simulink model "power_motordrive_PMSM_FOC"  (R2021a)
settings: Solver=FixedStepDiscrete  StartTime=0.0  StopTime=0.8  RelTol=1e-3  EnableMultiTasking=on
PreLoadFcn:
  |  power_motordrive_PMSM_FOC_data
InitFcn:
  | power_motordrive_PMSM_FOC_data
values from neighbouring files (symbols this model uses):
  Rs = 0.02    [foc_model_Initialization.m]
undefined symbols (not defined in the file or in its folder): DiscIntNeverNeededParam, F, Fsw, gcbh, J, Ki_Ireg, Ki_wreg, Kp_Ireg, Kp_wreg, Limit_Ireg, Limit_wreg, p, sps_rtmsupport, Ts, Vdc_nom
libraries: simulink x6, spsStairGeneratorLib x2, spsSecondOrderFilterLib x2, spsPermanentMagnetSynchronousMachineLib x1, spsDCVoltageSourceLib x1, spsdq0toabcLib x1, spsabctodq0Lib x1, spsPowerdq0InstantaneousLib x1, spsThreePhaseVIMeasurementLib x1, spsTwoLevelConverterLib x1, spspowerguiLib x1
settings Model: SimulationMode=accelerator  Creator=The MathWorks, Inc.  LastModifiedBy=Hidayet
settings SolverCC: AlgebraicLoopSolver=TrustRegion
settings DataIOCC: SaveOutput=off  SignalLogging=off  DSMLogging=off  SaveTime=off  ReturnWorkspaceOutputs=off
settings DebuggingCC: SFMachineParentedDataDiag=warning

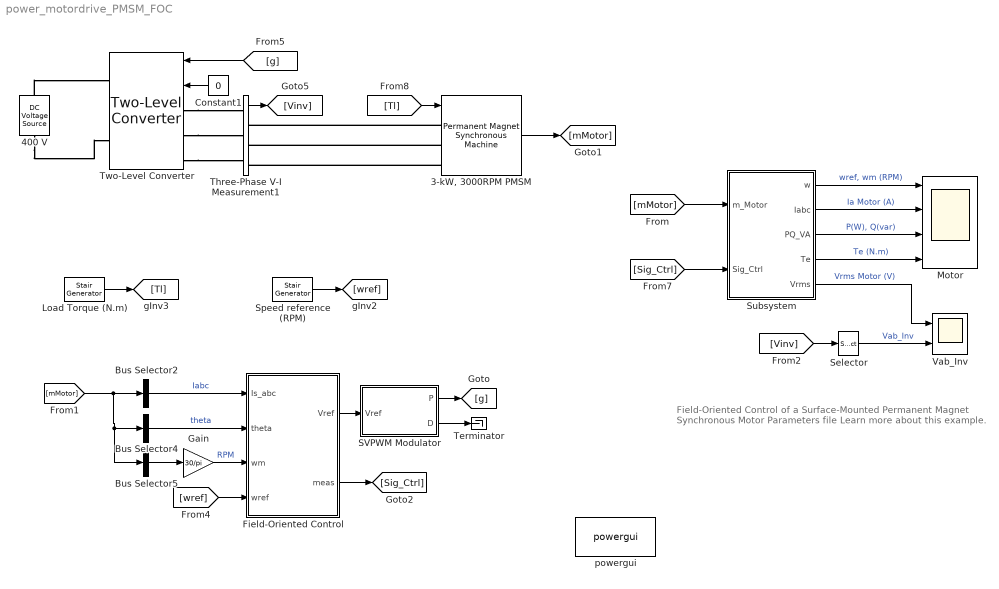
== system power_motordrive_PMSM_FOC ==
  note: Field-Oriented Control of a Surface-Mounted
      | Permanent Magnet Synchronous Motor
      | Parameters file
      |
      | Learn more about this example.
  "3-kW, 3000RPM PMSM" : spsPermanentMagnetSynchronousMachineLib/Permanent Magnet Synchronous Machine  NbPhases=3  FluxDistribution=Sinusoidal  RotorType=Round  MechanicalLoad=Torque Tm  PresetModel=No  ShowDetailedParameters=on  MeasurementBus=off  Resistance=Rs  Inductance=8.5e-3  dqInductances=[8.5e-3,8.5e-3]  La=La  MachineConstant=Flux linkage established by magnets (V.s)  Flux=lambda  VoltageCst=95.2245  TorqueCst=0.7875  Flat=120  Mechanical=[J F p 0]  PolePairs=4  InitialConditions=[0,0, 0,0]  InitialConditions5ph=[0 0 0 0 0 0]  RefAngle=90 degrees behind phase A axis (modified Park)  IterativeDiscreteModel=Trapezoidal robust  TsBlock=Ts  TsPowergui=0
  400 V : spsDCVoltageSourceLib/DC Voltage Source  Amplitude=Vdc_nom  Measurements=None
  Bus Selector2 : BusSelector  OutputSignals=Stator current is_a (A),Stator current is_b (A),Stator current is_c (A)  OutputAsBus=on
  Bus Selector4 : BusSelector  OutputSignals=Rotor angle thetam (rad)  OutputAsBus=on
  Bus Selector5 : BusSelector  OutputSignals=Rotor speed wm (rad/s)  OutputAsBus=on
  Constant1 : Constant  Value=0
  Field-Oriented Control : Subsystem  DialogController=POWERSYS.PowerSysDialog  LoadFcn=sps_rtmsupport('LoadFcn',gcbh);  StartFcn=sps_rtmsupport('StartFcn',gcbh);  StopFcn=sps_rtmsupport('StopFcn',gcbh);  mask(Field-Oriented Controller (FOC) of a PMSM drive){Kp_wreg=Kp_wreg, Ki_wreg=Ki_wreg, Limit_wreg=Limit_wreg, Kp_Ireg=Kp_Ireg, Ki_Ireg=Ki_Ireg, Limits_Ireg=Limit_Ireg, p=p, Ts=Ts}
      mask prompts: Kp_wreg "Proportional gain"; Ki_wreg "Integral gain"; Limit_wreg "Output (current) limit"; Kp_Ireg "Proportional gain"; Ki_Ireg "Integral gain"; Limits_Ireg "Output limit"; p "Number of pole pairs:"; Ts "Sample time (s)"
      settings: AttributesFormatString=\n  CopyFcn=sps_rtmsupport('CopyFcn',gcbh); powericon('psbloadfunction',gcbh,'gotofrom','UpdateGotoTag');  DeleteFcn=sps_rtmsupport('DeleteFcn',gcbh);  UndoDeleteFcn=sps_rtmsupport('UndoDeleteFcn',gcbh);  ModelCloseFcn=sps_rtmsupport('ModelCloseFcn',gcbh);  PreSaveFcn=sps_rtmsupport('PreSaveFcn',gcbh);  PostSaveFcn=sps_rtmsupport('PostSaveFcn',gcbh);  NameChangeFcn=sps_rtmsupport('NameChangeFcn',gcbh);  PreCopyFcn=sps_rtmsupport('PreCopyFcn',gcbh);  OpenFcn=sps_rtmsupport('OpenFcn',gcbh, [-1 2 -3 4 5 6 7 17 22 23]);  CloseFcn=sps_rtmsupport('CloseFcn',gcbh);  PreDeleteFcn=sps_rtmsupport('PreDeleteFcn',gcbh);
      mask Help: helpview(psbhelp);
      mask DialogControl Container11 Prompt: Control parameters
      mask DialogControl Container12 Prompt: Speed regulator
      mask DialogControl Container8 Prompt: Current regulators
  Gain : Gain  Gain=30/pi
  Load Torque (N.m) : spsStairGeneratorLib/Stair Generator  t=[0, 0.65]  e=[0,-8]  Ts=Ts
  Motor : Scope  NumInputPorts=4
  SVPWM Modulator : Subsystem  DialogController=POWERSYS.PowerSysDialog  LoadFcn=sps_rtmsupport('LoadFcn', gcbh);  StartFcn=sps_rtmsupport('StartFcn', gcbh);  StopFcn=sps_rtmsupport('StopFcn', gcbh);  mask(Unified PWM Modulator for a 2-level, 3-phase converter){PWMmethod=Space Vector PWM (SVPWM) with pulse averaging, Fsw=Fsw, Ts=Ts}
      mask prompts: PWMmethod "PWM method"; Fsw "Switching frequency (Hz):"; Ts "Sample time (s):"
      mask help:
      | Generate pulses for PWM-controlled two-level, three-phase power electronics converter with pulse averaging capability.
      |
      | The pulses generation can be perform using one of the following Pulse-Width Modulation (PWM) methods:
      | 1. Sinusoidal PWM (SPWM)
      | 2. Sinusoidal PWM (SPWM) with pulse averaging
      | 3. Space Vector PWM (SVPWM)
      | 4. Space Vector PWM (SVPWM) with pulse averaging
      | 5. 30 degrees discontinuous PWM
      |
      | When a PWM method with pulse averaging is selected, the output pulses are averaged over one sample time. (Pulses value will range from 0 to 1)
      mask init:
      | switch PWMmethod
      |     case 1 % SPWM
      |         ZeroOrderHold_Ts=-1;
      |         Pavg=0;
      |     case 2 % SPWM with pulse averaging
      |         ZeroOrderHold_Ts=-1;
      |         Pavg=1;
      |     case 3  % SVPWM
      |         ZeroOrderHold_Ts=-1;
      |         Pavg=0;
      |     case 4  % SVPWM with pulse averaging
      |         ZeroOrderHold_Ts=-1;
      |         Pavg=1;
      |     case 5  % 30 degrees discontinuous PWM
      |         ZeroOrderHold_Ts=1/Fsw/2;
      |         Pavg=0;
      | end
      settings: CopyFcn=sps_rtmsupport('CopyFcn', gcbh);  DeleteFcn=sps_rtmsupport('DeleteFcn', gcbh);  UndoDeleteFcn=sps_rtmsupport('UndoDeleteFcn', gcbh);  ModelCloseFcn=sps_rtmsupport('ModelCloseFcn', gcbh);  PreSaveFcn=sps_rtmsupport('PreSaveFcn', gcbh);  PostSaveFcn=sps_rtmsupport('PostSaveFcn', gcbh);  NameChangeFcn=sps_rtmsupport('NameChangeFcn', gcbh);  PreCopyFcn=sps_rtmsupport('PreCopyFcn', gcbh);  OpenFcn=sps_rtmsupport('OpenFcn', gcbh, [1]);  CloseFcn=sps_rtmsupport('CloseFcn', gcbh);  PreDeleteFcn=sps_rtmsupport('PreDeleteFcn', gcbh);
      mask TypeOptions PWMmethod: Sinusoidal PWM (SPWM) | Sinusoidal PWM (SPWM) wirh pulse averaging | Space Vector PWM (SVPWM) | Space Vector PWM (SVPWM) with pulse averaging | 30 degrees discontinuous PWM
  Selector : Selector  InputPortWidth=3  IndexOptions=Index vector (dialog)  Indices=1  OutputSizes=1
  Speed reference (RPM) : spsStairGeneratorLib/Stair Generator  t=[0, 0.25]  e=[2000, -2800]  Ts=Ts
  Subsystem : Subsystem
  Terminator : Terminator
  Three-Phase V-I Measurement1 : spsThreePhaseVIMeasurementLib/Three-Phase V-I Measurement  VoltageMeasurement=phase-to-phase  SetLabelV=off  LabelV=Vabc  Vpu=off  VpuLL=off  CurrentMeasurement=no  SetLabelI=off  LabelI=Iabc  Ipu=off  Pbase=100e6  Vbase=500e3  OutputType=Complex  PhasorSimulation=off  PSBequivalent=0
  Two-Level Converter : spsTwoLevelConverterLib/Two-Level Converter  ModelType=Switching function  Ron=1e-3  Rs=1e6  Cs=inf  Vforward=[0,0]  Ron_Diode=1e-3  Rs_Diode=1e6  Cs_Diode=inf  Vf_Diode=0  Rs_CurrentSource=inf
      settings: SourceProductBaseCode=PS
  Vab_Inv : Scope  NumInputPorts=2
  powergui : spspowerguiLib/powergui  Priority=1  SimulationMode=Discrete  SampleTime=Ts  frequency=60  Iterations=50  frequencyindice=0  Pbase=100e6  ErrMax=1e-4  UnitsV=kV  UnitsW=MW  buscounter=0  FunctionMessages=off  echomessages=off  EnableUseOfTLC=off  CurrentSourceSwitches=off  DisableSnubberDevices=off  DisableRonSwitches=off  DisableVfSwitches=off  DisplayEquations=off  AutomaticDiscreteSolvers=off  SolverType=Tustin/Backward Euler (TBE)  Interpol=off  ExternalGateDelay=off  methode=off  Ts=100  x0status=blocks  SPID=on  SwTol=0  HookPort=off  NonlinearTolerance=1e-4  nMaxIteration=100  ContinueOnMaxIteration=off  RestoreLinks=warning  ResistiveCurrentMeasurement=off  Frange=[0:2:500]  Ylog=off  Xlog=on  ShowGrid=off  save=off  variable=ZData  structure=Scope_Compare  ZoomFFT=off  StartTime=0.75  cycles=1  DisplayStyle=1  fundamental=100  FreqAxis=off  MaxFrequency=25000  frequencyindicesteady=1  RmsSteady=1  display=off
  wires:
  Subsystem/5(Vrms) -> Vab_Inv/1  "Vrms Motor (V)"
  Selector/1 -> Vab_Inv/2  "Vab_Inv"
  Subsystem/4(Te) -> Motor/4  "Te (N.m)"
  Field-Oriented Control/1(Vref) -> SVPWM Modulator/1(Vref)
  Field-Oriented Control/2(meas) -> [Sig_Ctrl]
  [Vinv] -> Selector/1
  Subsystem/1(w) -> Motor/1  "wref, wm (RPM)"
  Subsystem/2(Iabc) -> Motor/2  "Ia Motor (A)"
  Subsystem/3(PQ_VA) -> Motor/3  "P(W), Q(var)"
  [mMotor] -> Subsystem/1(m_Motor)
  [Sig_Ctrl] -> Subsystem/2(Sig_Ctrl)
  [wref] -> Field-Oriented Control/4(wref)
  [mMotor] -> Bus Selector2/1, Bus Selector4/1, Bus Selector5/1
  Bus Selector2/1 -> Field-Oriented Control/1(Is_abc)  "Iabc"
  "3-kW, 3000RPM PMSM"/1 -> [mMotor]
  Constant1/1 -> Two-Level Converter/2
  Three-Phase V-I Measurement1/1 -> [Vinv]
  [Tl] -> "3-kW, 3000RPM PMSM"/1
  [g] -> Two-Level Converter/1
  Speed reference (RPM)/1 -> [wref]
  Load Torque (N.m)/1 -> [Tl]
  Bus Selector5/1 -> Gain/1
  Gain/1 -> Field-Oriented Control/3(wm)  "RPM"
  Bus Selector4/1 -> Field-Oriented Control/2(theta)  "theta"
  SVPWM Modulator/1(P) -> [g]
  SVPWM Modulator/2(D) -> Terminator/1
  connections:
  400 V/RConn1 -- Two-Level Converter/RConn1
  "3-kW, 3000RPM PMSM"/LConn1 -- Three-Phase V-I Measurement1/RConn1
  Two-Level Converter/LConn3 -- Three-Phase V-I Measurement1/LConn3
  "3-kW, 3000RPM PMSM"/LConn2 -- Three-Phase V-I Measurement1/RConn2
  Two-Level Converter/LConn1 -- Three-Phase V-I Measurement1/LConn1
  Two-Level Converter/LConn2 -- Three-Phase V-I Measurement1/LConn2
  400 V/LConn1 -- Two-Level Converter/RConn2
  "3-kW, 3000RPM PMSM"/LConn3 -- Three-Phase V-I Measurement1/RConn3

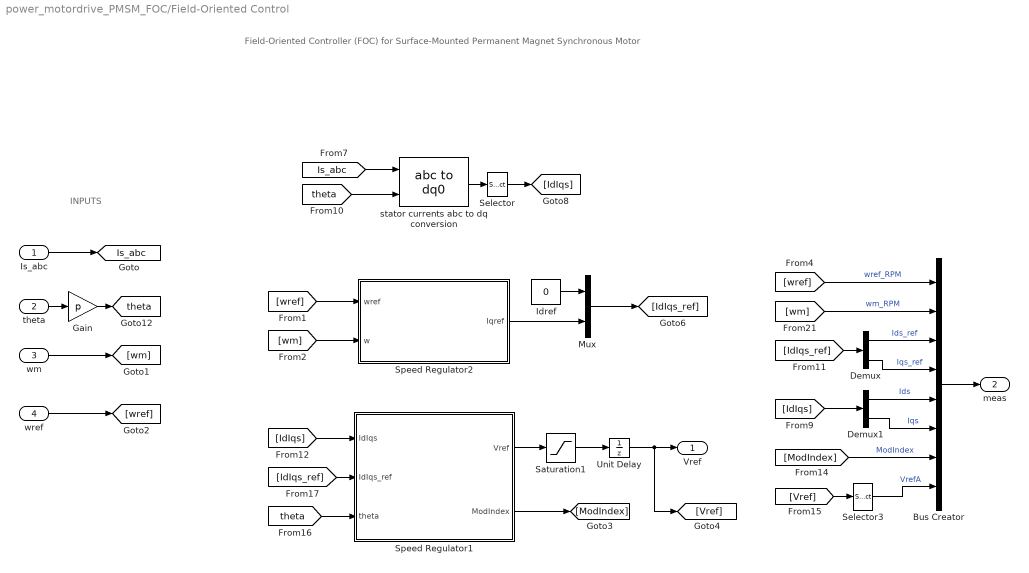
== system power_motordrive_PMSM_FOC/Field-Oriented Control ==
  note: INPUTS
  note: Field-Oriented Controller (FOC)
      | for
      | Surface-Mounted Permanent Magnet Synchronous Motor
  Is_abc : Inport  PortDimensions=3
  theta : Inport  Port=2  PortDimensions=1
  wm : Inport  Port=3  PortDimensions=1
  wref : Inport  Port=4  PortDimensions=1
  Bus Creator : BusCreator  Inputs=8
  Demux : Demux  Outputs=2
  Demux1 : Demux  Outputs=2
  Gain : Gain  Gain=p
  Idref : Constant  Value=0  SampleTime=Ts
  Mux : Mux  Inputs=2
  Saturation1 : Saturate  UpperLimit=2/sqrt(3)  LowerLimit=-2/sqrt(3)
  Selector : Selector  InputPortWidth=3  IndexOptions=Index vector (dialog)  Indices=[1 2]  OutputSizes=1
  Selector3 : Selector  InputPortWidth=3  IndexOptions=Index vector (dialog)  Indices=1  OutputSizes=1
  Speed Regulator1 : Subsystem  DialogController=POWERSYS.PowerSysDialog  mask(Current Regulators){Kp=Kp_Ireg, Ki=Ki_Ireg, Limits=Limits_Ireg, Init=0, Ts=Ts}
      mask prompts: Kp "Proportional gain (Kp):"; Ki "Integral gain (Ki):"; Limits "Output limits"; Init "Output initial value:"; Ts "Sample time:"
      mask help: This block implements two current regulators (Id & Iq) using anti-windup PI controllers.
      mask Display: disp('Current\nRegulators');
  Speed Regulator2 : Subsystem  DialogController=POWERSYS.PowerSysDialog  mask(Speed Regulator){Kp=Kp_wreg, Ki=Ki_wreg, Limit_wreg=Limit_wreg, Init=0, Ts=Ts}
      mask prompts: Kp "Proportional gain (Kp):"; Ki "Integral gain (Ki):"; Limit_wreg "Output limits"; Init "Output initial value:"; Ts "Sample time:"
      mask help: This block implements a speed regulator using an ant-windup PI controller.
      mask Display: disp('Speed\nRegulator');
  Unit Delay : UnitDelay  SampleTime=-1  HasFrameUpgradeWarning=on
  stator currents abc to dq conversion : spsabctodq0Lib/abc to dq0  Alignment=90 degrees behind phase A axis
  Vref : Outport  PortDimensions=3
  meas : Outport  Port=2
  tag scope: Is_abc=global, theta=global
  wires:
  Gain/1 -> [theta]
  Selector3/1 -> Bus Creator/8  "VrefA"
  [ModIndex] -> Bus Creator/7  "ModIndex"
  Mux/1 -> [IdIqs_ref]
  [IdIqs_ref] -> Speed Regulator1/2(IdIqs_ref)
  Idref/1 -> Mux/1
  Speed Regulator2/1(Iqref) -> Mux/2
  wref/1 -> [wref]
  theta/1 -> Gain/1
  Saturation1/1 -> Unit Delay/1
  [Vref] -> Selector3/1
  Speed Regulator1/2(ModIndex) -> [ModIndex]
  [IdIqs] -> Demux1/1
  Demux1/2 -> Bus Creator/6  "Iqs"
  Demux1/1 -> Bus Creator/5  "Ids"
  [IdIqs_ref] -> Demux/1
  Demux/2 -> Bus Creator/4  "Iqs_ref"
  Demux/1 -> Bus Creator/3  "Ids_ref"
  [wm] -> Bus Creator/2  "wm_RPM"
  [wref] -> Bus Creator/1  "wref_RPM"
  [IdIqs] -> Speed Regulator1/1(IdIqs)
  [theta] -> Speed Regulator1/3(theta)
  Is_abc/1 -> [Is_abc]
  Speed Regulator1/1(Vref) -> Saturation1/1
  stator currents abc to dq conversion/1 -> Selector/1
  [theta] -> stator currents abc to dq conversion/2
  [wm] -> Speed Regulator2/2(w)
  [wref] -> Speed Regulator2/1(wref)
  [Is_abc] -> stator currents abc to dq conversion/1
  Selector/1 -> [IdIqs]
  Unit Delay/1 -> [Vref], Vref/1
  Bus Creator/1 -> meas/1
  wm/1 -> [wm]

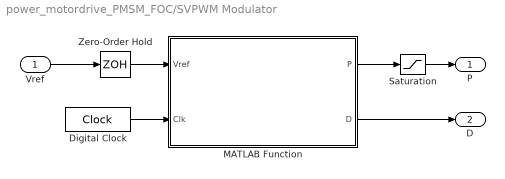
== system power_motordrive_PMSM_FOC/SVPWM Modulator ==
  Vref : Inport  PortDimensions=3  SampleTime=Ts
  Digital Clock : DigitalClock  SampleTime=Ts
  MATLAB Function : MATLAB Function  TreatAsAtomicUnit=on
  Saturation : Saturate  UpperLimit=1  LowerLimit=0
  Zero-Order Hold : ZeroOrderHold  SampleTime=ZeroOrderHold_Ts
  P : Outport  PortDimensions=6  SampleTime=Ts  VectorParamsAs1DForOutWhenUnconnected=off
  D : Outport  Port=2  PortDimensions=3  SampleTime=Ts  VectorParamsAs1DForOutWhenUnconnected=off
  wires:
  MATLAB Function/2(D) -> D/1
  MATLAB Function/1(P) -> Saturation/1
  Vref/1 -> Zero-Order Hold/1
  Saturation/1 -> P/1
  Digital Clock/1 -> MATLAB Function/2(Clk)
  Zero-Order Hold/1 -> MATLAB Function/1(Vref)

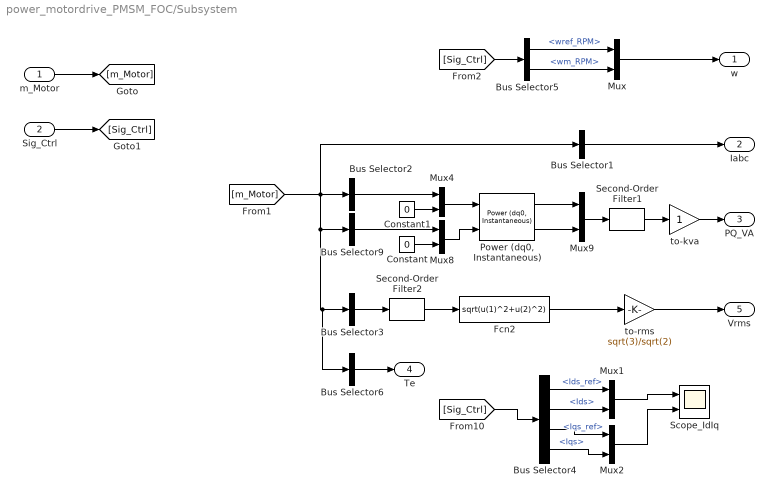
== system power_motordrive_PMSM_FOC/Subsystem ==
  m_Motor : Inport
  Sig_Ctrl : Inport  Port=2
  Bus Selector1 : BusSelector  OutputSignals=Stator current is_a (A),Stator current is_b (A),Stator current is_c (A)  OutputAsBus=on
  Bus Selector2 : BusSelector  OutputSignals=Stator voltage Vs_d (V),Stator voltage Vs_q (V)  OutputAsBus=on
  Bus Selector3 : BusSelector  OutputSignals=Stator voltage Vs_d (V),Stator voltage Vs_q (V)  OutputAsBus=on
  Bus Selector4 : BusSelector  OutputSignals=Ids_ref,Ids,Iqs_ref,Iqs
  Bus Selector5 : BusSelector  OutputSignals=wref_RPM,wm_RPM
  Bus Selector6 : BusSelector  OutputSignals=Electromagnetic torque Te (N*m)  OutputAsBus=on
  Bus Selector9 : BusSelector  OutputSignals=Stator current is_d (A),Stator current is_q (A)  OutputAsBus=on
  Constant : Constant  Value=0
  Constant1 : Constant  Value=0
  Fcn2 : Fcn  Expr=sqrt(u(1)^2+u(2)^2)
  Mux{,1..2,9} (4 alike) : Mux  Inputs=2
  Mux4 : Mux  Inputs=[2, 1]
  Mux8 : Mux  Inputs=[2, 1]
  "Power (dq0, Instantaneous)" : spsPowerdq0InstantaneousLib/Power (dq0, Instantaneous)
      settings: SourceProductBaseCode=PS
  Scope_IdIq : Scope  NumInputPorts=2
  Second-Order Filter1 : spsSecondOrderFilterLib/Second-Order Filter  FilterType=Lowpass  Fo=80  Zeta=1  Ts=Ts  Initialize=off  Vac_Init="[0,  0,  60]"  Vdc_Init=0  PlotResponse=off  FreqRange=[0, 500, 1]
      settings: SourceProductBaseCode=PS
  Second-Order Filter2 : spsSecondOrderFilterLib/Second-Order Filter  FilterType=Lowpass  Fo=120  Zeta=1  Ts=Ts  Initialize=off  Vac_Init="[0,  0,  60]"  Vdc_Init=0  PlotResponse=off  FreqRange=[0, 500, 1]
      settings: SourceProductBaseCode=PS
  to-kva : Gain
  to-rms : Gain  Gain=sqrt(3)/sqrt(2)
  w : Outport
  Iabc : Outport  Port=2
  PQ_VA : Outport  Port=3
  Te : Outport  Port=4
  Vrms : Outport  Port=5
  wires:
  Bus Selector6/1 -> Te/1
  Mux2/1 -> Scope_IdIq/2
  Mux1/1 -> Scope_IdIq/1
  Bus Selector4/4 -> Mux2/2  "<Iqs>"
  Bus Selector4/3 -> Mux2/1  "<Iqs_ref>"
  Bus Selector4/2 -> Mux1/2  "<Ids>"
  Bus Selector4/1 -> Mux1/1  "<Ids_ref>"
  Bus Selector1/1 -> Iabc/1
  Bus Selector5/2 -> Mux/2  "<wm_RPM>"
  Bus Selector5/1 -> Mux/1  "<wref_RPM>"
  [Sig_Ctrl] -> Bus Selector5/1
  [Sig_Ctrl] -> Bus Selector4/1
  Mux/1 -> w/1
  Mux8/1 -> "Power (dq0, Instantaneous)"/2
  Second-Order Filter2/1 -> Fcn2/1
  Fcn2/1 -> to-rms/1
  to-kva/1 -> PQ_VA/1
  to-rms/1 -> Vrms/1
  Second-Order Filter1/1 -> to-kva/1
  Mux9/1 -> Second-Order Filter1/1
  "Power (dq0, Instantaneous)"/1 -> Mux9/1
  Bus Selector2/1 -> Mux4/1
  "Power (dq0, Instantaneous)"/2 -> Mux9/2
  Constant/1 -> Mux8/2
  Bus Selector9/1 -> Mux8/1
  Constant1/1 -> Mux4/2
  Bus Selector3/1 -> Second-Order Filter2/1
  Mux4/1 -> "Power (dq0, Instantaneous)"/1
  [m_Motor] -> Bus Selector3/1, Bus Selector6/1, Bus Selector9/1, Bus Selector1/1, Bus Selector2/1
  m_Motor/1 -> [m_Motor]
  Sig_Ctrl/1 -> [Sig_Ctrl]

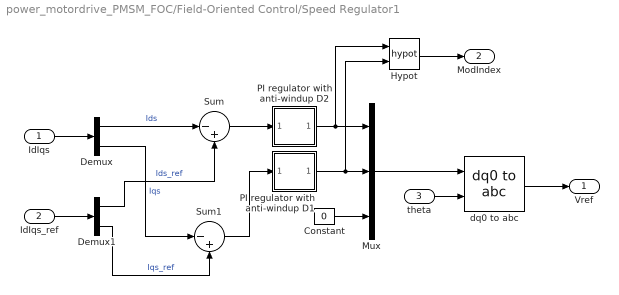
== system power_motordrive_PMSM_FOC/Field-Oriented Control/Speed Regulator1 ==
  IdIqs : Inport  PortDimensions=2
  IdIqs_ref : Inport  Port=2  PortDimensions=2
  theta : Inport  Port=3  PortDimensions=1
  Constant : Constant  Value=0
  Demux : Demux  Outputs=2
  Demux1 : Demux  Outputs=2
  Hypot : Math  Operator=hypot  SaturateOnIntegerOverflow=on
  Mux : Mux  Inputs=3
  PI regulator with anti-windup D1 : Subsystem  DialogController=POWERSYS.PowerSysDialog  mask(Discrete PI Controller){Kp=Kp, Ki=Ki, Par_Limits=[Limits -Limits], Init=0, Ts=Ts}
      mask prompts: Kp "Proportional gain (Kp):"; Ki "Integral gain (Ki):"; Par_Limits "Output limits: [ Upper   Lower ]"; Init "Output initial value:"; Ts "Sample time:"
      mask help: This block implements a discrete PI controller.
      mask init:
      | UpperLimit=Par_Limits(1);
      | LowerLimit=Par_Limits(2);
      | power_initmask();
      mask Help: This block is part of a subset of blocks in the Extras library that does not have documentation associated with it, other than the block mask description.
      mask Display: disp('PI');
  PI regulator with anti-windup D2 : Subsystem  DialogController=POWERSYS.PowerSysDialog  mask(Discrete PI Controller){Kp=Kp, Ki=Ki, Par_Limits=[Limits -Limits], Init=0, Ts=Ts}
      mask prompts: Kp "Proportional gain (Kp):"; Ki "Integral gain (Ki):"; Par_Limits "Output limits: [ Upper   Lower ]"; Init "Output initial value:"; Ts "Sample time:"
      mask help: This block implements a discrete PI controller.
      mask init:
      | UpperLimit=Par_Limits(1);
      | LowerLimit=Par_Limits(2);
      | power_initmask();
      mask Help: This block is part of a subset of blocks in the Extras library that does not have documentation associated with it, other than the block mask description.
      mask Display: disp('PI');
  Sum : Sum  Inputs=|-+
  Sum1 : Sum  Inputs=|-+
  dq0 to abc : spsdq0toabcLib/dq0 to abc  Alignment=90 degrees behind phase A axis
  Vref : Outport
  ModIndex : Outport  Port=2
  wires:
  Hypot/1 -> ModIndex/1
  dq0 to abc/1 -> Vref/1
  Demux1/1 -> Sum/2  "Ids_ref"
  Demux/1 -> Sum/1  "Ids"
  Demux1/2 -> Sum1/2  "Iqs_ref"
  IdIqs_ref/1 -> Demux1/1
  IdIqs/1 -> Demux/1
  PI regulator with anti-windup D2/1(Out) -> Mux/1, Hypot/1
  Sum/1 -> PI regulator with anti-windup D2/1(Error)
  PI regulator with anti-windup D1/1(Out) -> Mux/2, Hypot/2
  Constant/1 -> Mux/3
  Sum1/1 -> PI regulator with anti-windup D1/1(Error)
  Mux/1 -> dq0 to abc/1
  theta/1 -> dq0 to abc/2
  Demux/2 -> Sum1/1  "Iqs"

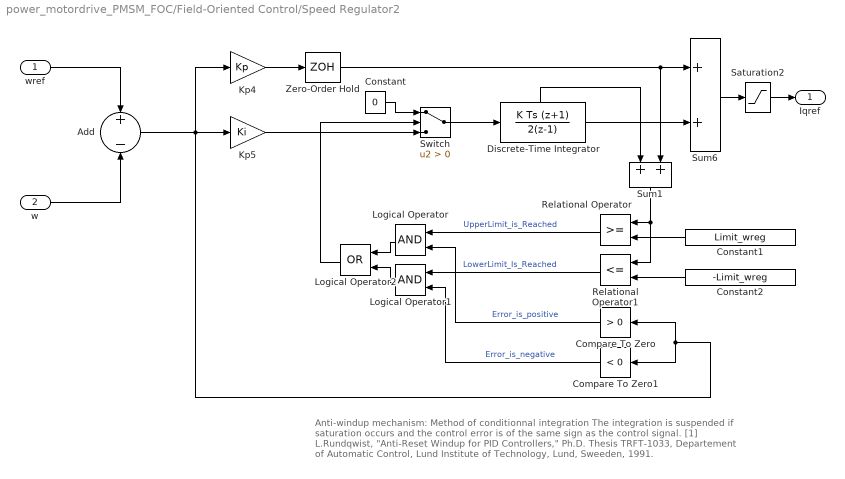
== system power_motordrive_PMSM_FOC/Field-Oriented Control/Speed Regulator2 ==
  note: Anti-windup mechanism: Method of conditionnal integration
      |
      | The integration is suspended if saturation occurs and the
      | control error is of the same sign as the control signal.
      |
      | [1] L.Rundqwist, "Anti-Reset Windup for PID Controllers," Ph.D. Thesis TRFT-1033,
      | Departement of Automatic Control, Lund Institute of Technology, Lund, Sweeden, 1991.
  wref : Inport  PortDimensions=1
  w : Inport  Port=2  PortDimensions=1
  Add : Sum  Inputs=+|-
  Compare To Zero : simulink/Logic and Bit Operations/Compare To Zero  relop=>  OutDataTypeStr=uint8  ZeroCross=off
  Compare To Zero1 : simulink/Logic and Bit Operations/Compare To Zero  relop=<  OutDataTypeStr=uint8  ZeroCross=off
  Constant : Constant  Value=0
  Constant1 : Constant  Value=Limit_wreg
  Constant2 : Constant  Value=-Limit_wreg
  Discrete-Time Integrator : DiscreteIntegrator  IntegratorMethod=Integration: Trapezoidal  InitialCondition=Init  SampleTime=Ts  LimitOutput=on  UpperSaturationLimit=Limit_wreg  LowerSaturationLimit=-Limit_wreg  ShowStatePort=on  ICPrevOutput=DiscIntNeverNeededParam  ICPrevScaledInput=DiscIntNeverNeededParam
  Kp4 : Gain  Gain=Kp  SaturateOnIntegerOverflow=on  SampleTime=Ts  OutDataTypeStr=Inherit: Same as input  ParamDataTypeStr=Inherit: Same as input
  Kp5 : Gain  Gain=Ki  SaturateOnIntegerOverflow=on  SampleTime=Ts  OutDataTypeStr=Inherit: Same as input  ParamDataTypeStr=Inherit: Same as input
  Logical Operator : Logic  AllPortsSameDT=off  OutDataTypeStr=boolean
  Logical Operator1 : Logic  AllPortsSameDT=off  OutDataTypeStr=boolean
  Logical Operator2 : Logic  Operator=OR  AllPortsSameDT=off  OutDataTypeStr=boolean
  Relational Operator : RelationalOperator  OutDataTypeStr=boolean  RndMeth=Nearest
  Relational Operator1 : RelationalOperator  Operator=<=  OutDataTypeStr=boolean  RndMeth=Nearest
  Saturation2 : Saturate  UpperLimit=Limit_wreg  LowerLimit=-Limit_wreg  SampleTime=Ts
  Sum1 : Sum  InputSameDT=on  SaturateOnIntegerOverflow=on  SampleTime=Ts  OutDataTypeStr=Inherit: Same as first input
  Sum6 : Sum  InputSameDT=on  SaturateOnIntegerOverflow=on  SampleTime=Ts  OutDataTypeStr=Inherit: Same as first input
  Switch : Switch  Criteria=u2 > Threshold
  Zero-Order Hold : ZeroOrderHold  SampleTime=Ts
  Iqref : Outport  SampleTime=Ts  InitialOutput=0  VectorParamsAs1DForOutWhenUnconnected=off
  wires:
  Kp5/1 -> Switch/3
  Switch/1 -> Discrete-Time Integrator/1
  Saturation2/1 -> Iqref/1
  Discrete-Time Integrator/1 -> Sum6/2
  Kp4/1 -> Zero-Order Hold/1
  Sum6/1 -> Saturation2/1
  Add/1 -> Compare To Zero/1, Compare To Zero1/1, Kp5/1, Kp4/1
  Compare To Zero1/1 -> Logical Operator1/2  "Error_is_negative"
  Logical Operator1/1 -> Logical Operator2/2
  Logical Operator/1 -> Logical Operator2/1
  Compare To Zero/1 -> Logical Operator/2  "Error_is_positive"
  Constant2/1 -> Relational Operator1/2
  Constant1/1 -> Relational Operator/2
  Relational Operator1/1 -> Logical Operator1/1  "LowerLimit_Is_Reached"
  Relational Operator/1 -> Logical Operator/1  "UpperLimit_is_Reached"
  Logical Operator2/1 -> Switch/2
  Sum1/1 -> Relational Operator/1, Relational Operator1/1
  Discrete-Time Integrator/State -> Sum1/1
  Zero-Order Hold/1 -> Sum6/1, Sum1/2
  Constant/1 -> Switch/1
  wref/1 -> Add/1
  w/1 -> Add/2

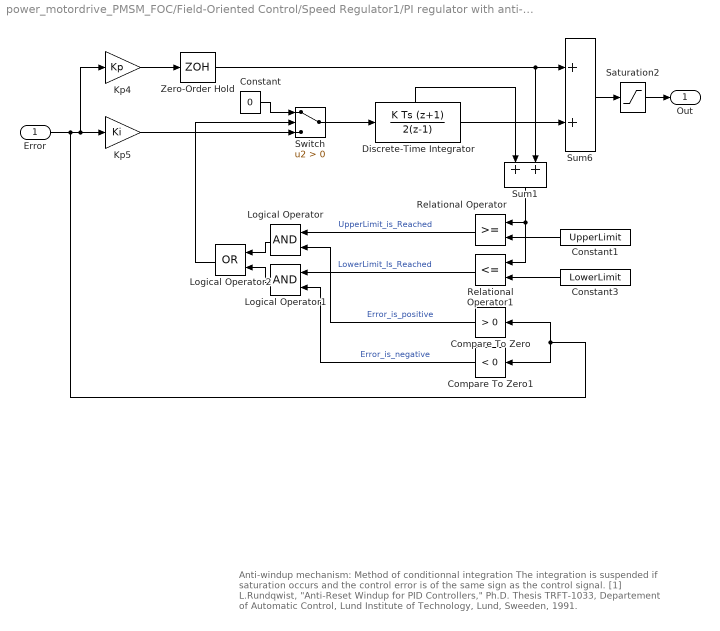
== system power_motordrive_PMSM_FOC/Field-Oriented Control/Speed Regulator1/PI regulator with anti-windup D1 ==
  note: Anti-windup mechanism: Method of conditionnal integration
      |
      | The integration is suspended if saturation occurs and the
      | control error is of the same sign as the control signal.
      |
      | [1] L.Rundqwist, "Anti-Reset Windup for PID Controllers," Ph.D. Thesis TRFT-1033,
      | Departement of Automatic Control, Lund Institute of Technology, Lund, Sweeden, 1991.
  Error : Inport  SampleTime=Ts
  Compare To Zero : simulink/Logic and Bit Operations/Compare To Zero  relop=>  OutDataTypeStr=uint8  ZeroCross=off
  Compare To Zero1 : simulink/Logic and Bit Operations/Compare To Zero  relop=<  OutDataTypeStr=uint8  ZeroCross=off
  Constant : Constant  Value=0
  Constant1 : Constant  Value=UpperLimit
  Constant3 : Constant  Value=LowerLimit
  Discrete-Time Integrator : DiscreteIntegrator  IntegratorMethod=Integration: Trapezoidal  InitialCondition=Init  SampleTime=Ts  LimitOutput=on  UpperSaturationLimit=UpperLimit  LowerSaturationLimit=LowerLimit  ShowStatePort=on  ICPrevOutput=DiscIntNeverNeededParam  ICPrevScaledInput=DiscIntNeverNeededParam
  Kp4 : Gain  Gain=Kp  SaturateOnIntegerOverflow=on  SampleTime=Ts  OutDataTypeStr=Inherit: Same as input  ParamDataTypeStr=Inherit: Same as input
  Kp5 : Gain  Gain=Ki  SaturateOnIntegerOverflow=on  SampleTime=Ts  OutDataTypeStr=Inherit: Same as input  ParamDataTypeStr=Inherit: Same as input
  Logical Operator : Logic  AllPortsSameDT=off  OutDataTypeStr=boolean
  Logical Operator1 : Logic  AllPortsSameDT=off  OutDataTypeStr=boolean
  Logical Operator2 : Logic  Operator=OR  AllPortsSameDT=off  OutDataTypeStr=boolean
  Relational Operator : RelationalOperator  OutDataTypeStr=boolean  RndMeth=Nearest
  Relational Operator1 : RelationalOperator  Operator=<=  OutDataTypeStr=boolean  RndMeth=Nearest
  Saturation2 : Saturate  UpperLimit=UpperLimit  LowerLimit=LowerLimit  SampleTime=Ts
  Sum1 : Sum  InputSameDT=on  SaturateOnIntegerOverflow=on  SampleTime=Ts  OutDataTypeStr=Inherit: Same as first input
  Sum6 : Sum  InputSameDT=on  SaturateOnIntegerOverflow=on  SampleTime=Ts  OutDataTypeStr=Inherit: Same as first input
  Switch : Switch  Criteria=u2 > Threshold
  Zero-Order Hold : ZeroOrderHold  SampleTime=Ts
  Out : Outport  SampleTime=Ts  InitialOutput=0
  wires:
  Constant/1 -> Switch/1
  Zero-Order Hold/1 -> Sum1/2, Sum6/1
  Discrete-Time Integrator/State -> Sum1/1
  Sum1/1 -> Relational Operator1/1, Relational Operator/1
  Logical Operator2/1 -> Switch/2
  Relational Operator/1 -> Logical Operator/1  "UpperLimit_is_Reached"
  Relational Operator1/1 -> Logical Operator1/1  "LowerLimit_Is_Reached"
  Constant1/1 -> Relational Operator/2
  Constant3/1 -> Relational Operator1/2
  Compare To Zero/1 -> Logical Operator/2  "Error_is_positive"
  Logical Operator/1 -> Logical Operator2/1
  Logical Operator1/1 -> Logical Operator2/2
  Compare To Zero1/1 -> Logical Operator1/2  "Error_is_negative"
  Error/1 -> Compare To Zero1/1, Compare To Zero/1, Kp4/1, Kp5/1
  Sum6/1 -> Saturation2/1
  Kp4/1 -> Zero-Order Hold/1
  Discrete-Time Integrator/1 -> Sum6/2
  Saturation2/1 -> Out/1
  Switch/1 -> Discrete-Time Integrator/1
  Kp5/1 -> Switch/3

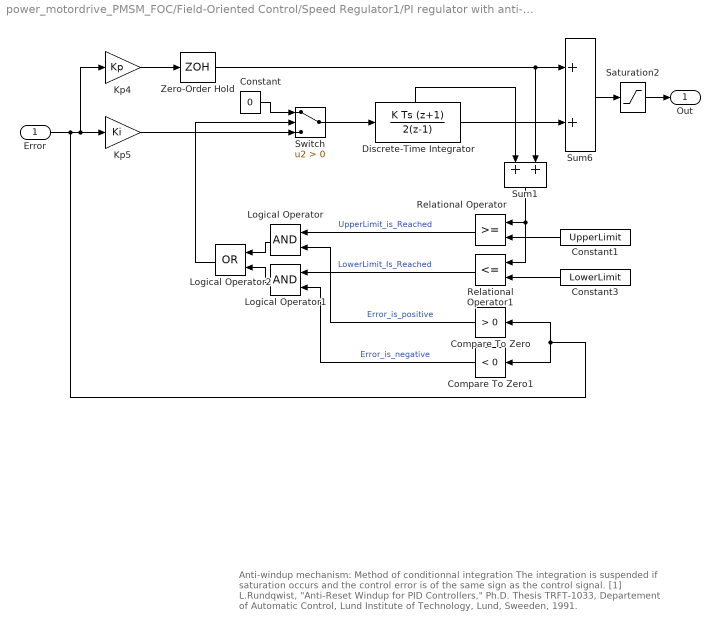
== system power_motordrive_PMSM_FOC/Field-Oriented Control/Speed Regulator1/PI regulator with anti-windup D2 ==
  note: Anti-windup mechanism: Method of conditionnal integration
      |
      | The integration is suspended if saturation occurs and the
      | control error is of the same sign as the control signal.
      |
      | [1] L.Rundqwist, "Anti-Reset Windup for PID Controllers," Ph.D. Thesis TRFT-1033,
      | Departement of Automatic Control, Lund Institute of Technology, Lund, Sweeden, 1991.
  Error : Inport  SampleTime=Ts
  Compare To Zero : simulink/Logic and Bit Operations/Compare To Zero  relop=>  OutDataTypeStr=uint8  ZeroCross=off
  Compare To Zero1 : simulink/Logic and Bit Operations/Compare To Zero  relop=<  OutDataTypeStr=uint8  ZeroCross=off
  Constant : Constant  Value=0
  Constant1 : Constant  Value=UpperLimit
  Constant3 : Constant  Value=LowerLimit
  Discrete-Time Integrator : DiscreteIntegrator  IntegratorMethod=Integration: Trapezoidal  InitialCondition=Init  SampleTime=Ts  LimitOutput=on  UpperSaturationLimit=UpperLimit  LowerSaturationLimit=LowerLimit  ShowStatePort=on  ICPrevOutput=DiscIntNeverNeededParam  ICPrevScaledInput=DiscIntNeverNeededParam
  Kp4 : Gain  Gain=Kp  SaturateOnIntegerOverflow=on  SampleTime=Ts  OutDataTypeStr=Inherit: Same as input  ParamDataTypeStr=Inherit: Same as input
  Kp5 : Gain  Gain=Ki  SaturateOnIntegerOverflow=on  SampleTime=Ts  OutDataTypeStr=Inherit: Same as input  ParamDataTypeStr=Inherit: Same as input
  Logical Operator : Logic  AllPortsSameDT=off  OutDataTypeStr=boolean
  Logical Operator1 : Logic  AllPortsSameDT=off  OutDataTypeStr=boolean
  Logical Operator2 : Logic  Operator=OR  AllPortsSameDT=off  OutDataTypeStr=boolean
  Relational Operator : RelationalOperator  OutDataTypeStr=boolean  RndMeth=Nearest
  Relational Operator1 : RelationalOperator  Operator=<=  OutDataTypeStr=boolean  RndMeth=Nearest
  Saturation2 : Saturate  UpperLimit=UpperLimit  LowerLimit=LowerLimit  SampleTime=Ts
  Sum1 : Sum  InputSameDT=on  SaturateOnIntegerOverflow=on  SampleTime=Ts  OutDataTypeStr=Inherit: Same as first input
  Sum6 : Sum  InputSameDT=on  SaturateOnIntegerOverflow=on  SampleTime=Ts  OutDataTypeStr=Inherit: Same as first input
  Switch : Switch  Criteria=u2 > Threshold
  Zero-Order Hold : ZeroOrderHold  SampleTime=Ts
  Out : Outport  SampleTime=Ts  InitialOutput=0
  wires:
  Kp5/1 -> Switch/3
  Switch/1 -> Discrete-Time Integrator/1
  Saturation2/1 -> Out/1
  Discrete-Time Integrator/1 -> Sum6/2
  Kp4/1 -> Zero-Order Hold/1
  Sum6/1 -> Saturation2/1
  Error/1 -> Kp5/1, Kp4/1, Compare To Zero/1, Compare To Zero1/1
  Compare To Zero1/1 -> Logical Operator1/2  "Error_is_negative"
  Logical Operator1/1 -> Logical Operator2/2
  Logical Operator/1 -> Logical Operator2/1
  Compare To Zero/1 -> Logical Operator/2  "Error_is_positive"
  Constant3/1 -> Relational Operator1/2
  Constant1/1 -> Relational Operator/2
  Relational Operator1/1 -> Logical Operator1/1  "LowerLimit_Is_Reached"
  Relational Operator/1 -> Logical Operator/1  "UpperLimit_is_Reached"
  Logical Operator2/1 -> Switch/2
  Sum1/1 -> Relational Operator/1, Relational Operator1/1
  Discrete-Time Integrator/State -> Sum1/1
  Zero-Order Hold/1 -> Sum6/1, Sum1/2
  Constant/1 -> Switch/1

== matlab function power_motordrive_PMSM_FOC/SVPWM Modulator/MATLAB Function ==
  data: Ts parameter; Fsw parameter; Vref input; P output; PWMmethod parameter; D output; Clk input; Pavg parameter
function [P, D]   = ...
    UnifiedPWMModulator_2Levelx(Ts, Fsw, Vref, PWMmethod, Clk, Pavg)
[P, D]   = ...
    unifiedPWMModulator2Level(Ts, Fsw, Vref, PWMmethod, Pavg, Clk);
